simulink model "pendulum_ctrl_sim_2"  (R2023a)
settings: Solver=VariableStepAuto  StartTime=0.0  StopTime=Tf_2  MaxStep=MaxStep  RelTol=RelTol
values from neighbouring files (symbols this model uses):
  A_ctrl = R_s_lti.A    [p60_pendulum_control.m]
  b = 0.05    [p60_pendulum_control.m]
  B_ctrl = R_s_lti.B    [p60_pendulum_control.m]
  C_ctrl = R_s_lti.C    [p60_pendulum_control.m]
  D_ctrl = R_s_lti.D    [p60_pendulum_control.m]
  g = 9.81    [p60_pendulum_control.m]
  l = 0.3    [p60_pendulum_control.m]
  M = 0.5    [p60_pendulum_control.m]
  theta_star_s = pi/3    (= 1.0471975512)    [p60_pendulum_control.m]
  x0_2 = [0; 0]    [p60_pendulum_control.m]
settings Model: Creator=alessandro  LastModifiedBy=admin
settings OptimizationCC: ReuseModelBlockBuffer=off

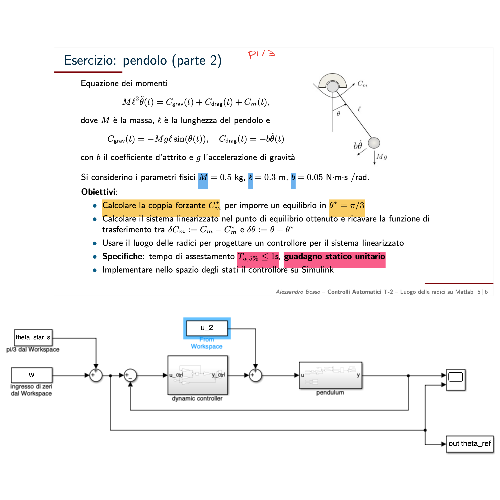
[thumbnail: Simulink's stored preview of the top-level diagram]
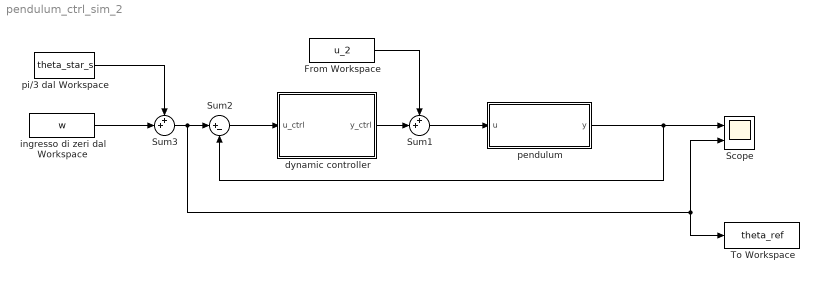
== system pendulum_ctrl_sim_2 ==
  From Workspace : FromWorkspace  VariableName=u_2
  Scope : Scope  NumInputPorts=2
  Sum1 : Sum  Inputs=++|
  Sum2 : Sum  Inputs=|+-
  Sum3 : Sum  Inputs=++|
  To Workspace : ToWorkspace  VariableName=theta_ref  SaveFormat=Timeseries  SampleTime=-1
  dynamic controller : Subsystem
  ingresso di zeri dal Workspace : FromWorkspace  VariableName=w
  pendulum : Subsystem
  pi/3 dal Workspace : Constant  Value=theta_star_s
  wires:
  Sum2/1 -> dynamic controller/1(u_ctrl)
  From Workspace/1 -> Sum1/1
  Sum1/1 -> pendulum/1(u)
  pendulum/1(y) -> Scope/1, Sum2/2
  Sum3/1 -> Scope/2, To Workspace/1, Sum2/1
  dynamic controller/1(y_ctrl) -> Sum1/2
  pi/3 dal Workspace/1 -> Sum3/1
  ingresso di zeri dal Workspace/1 -> Sum3/2

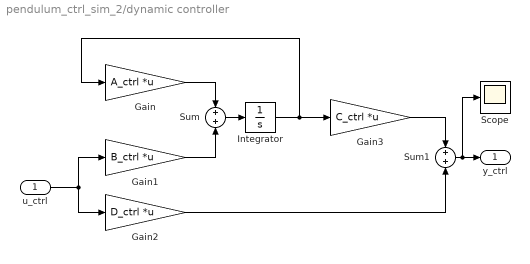
== system pendulum_ctrl_sim_2/dynamic controller ==
  u_ctrl : Inport
  Gain : Gain  Gain=A_ctrl  Multiplication=Matrix(K*u)
  Gain1 : Gain  Gain=B_ctrl  Multiplication=Matrix(K*u)
  Gain2 : Gain  Gain=D_ctrl  Multiplication=Matrix(K*u)
  Gain3 : Gain  Gain=C_ctrl  Multiplication=Matrix(K*u)
  Integrator : Integrator
  Scope : Scope
  Sum : Sum
  Sum1 : Sum
  y_ctrl : Outport
  wires:
  Sum/1 -> Integrator/1
  Gain/1 -> Sum/1
  u_ctrl/1 -> Gain1/1, Gain2/1
  Integrator/1 -> Gain3/1, Gain/1
  Gain1/1 -> Sum/2
  Sum1/1 -> Scope/1, y_ctrl/1
  Gain3/1 -> Sum1/1
  Gain2/1 -> Sum1/2

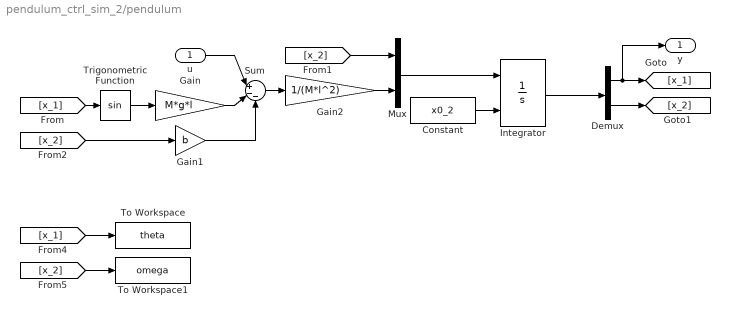
== system pendulum_ctrl_sim_2/pendulum ==
  u : Inport
  Constant : Constant  Value=x0_2
  Demux : Demux  Outputs=2
  Gain : Gain  Gain=M*g*l
  Gain1 : Gain  Gain=b
  Gain2 : Gain  Gain=1/(M*l^2)
  Integrator : Integrator  InitialConditionSource=external
  Mux : Mux  Inputs=2
  Sum : Sum  Inputs=|+--
  To Workspace : ToWorkspace  VariableName=theta  SaveFormat=Timeseries  SampleTime=-1
  To Workspace1 : ToWorkspace  VariableName=omega  SaveFormat=Timeseries  SampleTime=-1
  Trigonometric Function : Trigonometry
  y : Outport
  wires:
  [x_2] -> Gain1/1
  [x_1] -> To Workspace/1
  Mux/1 -> Integrator/1
  Sum/1 -> Gain2/1
  Demux/2 -> [x_2]
  Integrator/1 -> Demux/1
  [x_2] -> To Workspace1/1
  Demux/1 -> y/1, [x_1]
  Gain1/1 -> Sum/3
  Gain2/1 -> Mux/2
  [x_1] -> Trigonometric Function/1
  Constant/1 -> Integrator/2
  Gain/1 -> Sum/2
  Trigonometric Function/1 -> Gain/1
  [x_2] -> Mux/1
  u/1 -> Sum/1
